simulink model "steering_validation"  (R2018b)
settings: Solver=VariableStepAuto  StartTime=0.0  StopTime=10.0  RelTol=1e-3
values from neighbouring files (symbols this model uses):
  D_steering_position = 0    [report_gutman.m]    (also in steering_extract_data.m)
  I_steering_position = 30    [report_gutman.m]    (also in steering_extract_data.m = 0)
  K_feedforward_steering = 0    [report_gutman.m]    (also in steering_extract_data.m)
  num_tf_steering = [253.4]    [report_gutman.m]    (also in steering_extract_data.m)
  P_steering_position = 30    [report_gutman.m]    (also in steering_extract_data.m)
  Ts = 0.01    [plot_poles.m]    (also in report_gutman.m; steering_extract_data.m)
libraries: simulink_extras x4, simulink x2
settings Model: Creator=maximef  LastModifiedBy=maximef

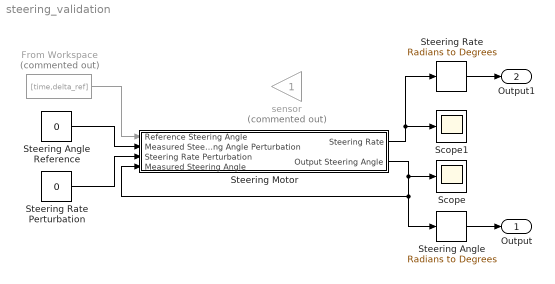
== system steering_validation ==
  From Workspace : FromWorkspace  Commented=on  VariableName=[time,delta_ref]  SampleTime=0
  Scope : Scope
  Scope1 : Scope
  Steering Angle : simulink_extras/Transformations/Radians to Degrees
  Steering Angle Reference : Constant  Value=0
  Steering Motor : Subsystem
  Steering Rate : simulink_extras/Transformations/Radians to Degrees
  Steering Rate Perturbation : Constant  Value=0
  sensor : Gain  Commented=on
  Output : Outport
  Output1 : Outport  Port=2
  wires:
  From Workspace/1 -> Steering Motor/1(Reference Steering Angle)
  Steering Motor/2(Output Steering Angle) -> Steering Angle/1, Steering Motor/4(Measured Steering Angle), Scope/1
  Steering Angle/1 -> Output/1
  Steering Rate Perturbation/1 -> Steering Motor/3(Steering Rate Perturbation)
  Steering Angle Reference/1 -> Steering Motor/2(Measured Steering Angle Perturbation)
  Steering Rate/1 -> Output1/1
  Steering Motor/1(Steering Rate) -> Scope1/1, Steering Rate/1

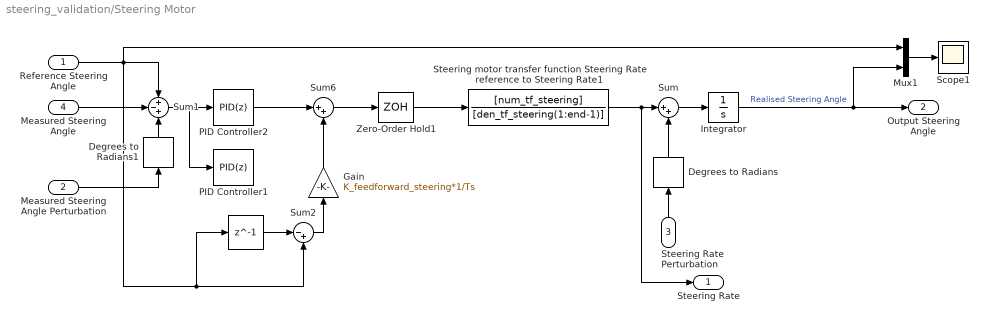
== system steering_validation/Steering Motor ==
  Reference Steering Angle : Inport
  Measured Steering Angle Perturbation : Inport  Port=2
  Steering Rate Perturbation : Inport  Port=3
  Measured Steering Angle : Inport  Port=4
  " " : Delay  DelayLength=1  SampleTime=Ts
  Degrees to Radians : simulink_extras/Transformations/Degrees to Radians
  Degrees to Radians1 : simulink_extras/Transformations/Degrees to Radians
  Gain : Gain  Gain=K_feedforward_steering*1/Ts
  Integrator : Integrator  InitialCondition=deg2rad(2)
  Mux1 : Mux  Inputs=2
  PID Controller1 : simulink/Continuous/PID Controller  Controller=PID  Form=Parallel  TimeDomain=Discrete-time  SampleTime=Ts  IntegratorMethod=Forward Euler  FilterMethod=Forward Euler  ControllerParametersSource=internal  P=P_steering_position  I=I_steering_position  D=D_steering_position  UseFilter=off  N=1  TunerSelectOption=Transfer Function Based (PID Tuner App)  InitialConditionSource=internal  InitialConditionForIntegrator=0  InitialConditionForFilter=0  DifferentiatorICPrevScaledInput=0  ExternalReset=none  TrackingMode=off  Kt=1  LimitOutput=off  UpperSaturationLimit=inf  LowerSaturationLimit=-inf  LinearizeAsGain=on  AntiWindupMode=none  Kb=1  POutMin=[]  POutMax=[]  IOutMin=[]  IOutMax=[]  DOutMin=[]  DOutMax=[]  NOutMin=[]  NOutMax=[]  SumOutMin=[]  SumOutMax=[]  SaturationOutMin=[]  SaturationOutMax=[]  PParamMin=[]  PParamMax=[]  IParamMin=[]  IParamMax=[]  DParamMin=[]  DParamMax=[]  NParamMin=[]  NParamMax=[]  KbParamMin=[]  KbParamMax=[]  KtParamMin=[]  KtParamMax=[]  KbOutMin=[]  KbOutMax=[]  KtOutMin=[]  KtOutMax=[]  IntegratorOutMin=[]  IntegratorOutMax=[]  FilterOutMin=[]  FilterOutMax=[]  SumI1OutMin=[]  SumI1OutMax=[]  SumI2OutMin=[]  SumI2OutMax=[]  SumI3OutMin=[]  SumI3OutMax=[]  SumI4OutMin=[]  SumI4OutMax=[]  SumDOutMin=[]  SumDOutMax=[]  DifferentiatorOutMin=[]  DifferentiatorOutMax=[]  FilterDiffOutCoefMin=[]  FilterDiffOutCoefMax=[]  ReciprocalOutMin=[]  ReciprocalOutMax=[]  SumDenOutMin=[]  SumDenOutMax=[]  SumNumOutMin=[]  SumNumOutMax=[]  DivideOutMin=[]  DivideOutMax=[]  IntegratorContinuousStateAttributes=''  IntegratorStateMustResolveToSignalObject=off  IntegratorRTWStateStorageClass=Auto  FilterContinuousStateAttributes=''  FilterStateMustResolveToSignalObject=off  FilterRTWStateStorageClass=Auto  ParallelPVariant=InternalParameters  IdealPVariant=Disabled  IVariant=InternalParameters  DVariant=InternalParameters  IntegratorVariant=Discrete  SatVariant=Disabled  AWVariant=Passthrough  PCopyVariant=Disabled  TRVariant=Disabled  FdbkBlocksVariant=Forward  IdealPFdbkVariant=Disabled  SatFdbkVariant=Disabled  DerivativeFilterVariant=Differentiator  NVariant=Passthrough  NCopyVariant=Disabled_SignalSpec  FilterICVariant=InternalICsDifferentiator  IntegratorICVariant=InternalICs  ExternalResetVariant=Disabled  TRSumVariant=Passthrough  SumFdbkVariant=Disabled  SumVariant=Sum_PID
  PID Controller2 : simulink/Continuous/PID Controller  Controller=PID  Form=Parallel  TimeDomain=Discrete-time  SampleTime=Ts  IntegratorMethod=Forward Euler  FilterMethod=Forward Euler  ControllerParametersSource=internal  P=0.1  I=0  D=0.04  UseFilter=off  N=1  TunerSelectOption=Transfer Function Based (PID Tuner App)  InitialConditionSource=internal  InitialConditionForIntegrator=0  InitialConditionForFilter=0  DifferentiatorICPrevScaledInput=0  ExternalReset=none  TrackingMode=off  Kt=1  LimitOutput=off  UpperSaturationLimit=inf  LowerSaturationLimit=-inf  LinearizeAsGain=on  AntiWindupMode=none  Kb=1  POutMin=[]  POutMax=[]  IOutMin=[]  IOutMax=[]  DOutMin=[]  DOutMax=[]  NOutMin=[]  NOutMax=[]  SumOutMin=[]  SumOutMax=[]  SaturationOutMin=[]  SaturationOutMax=[]  PParamMin=[]  PParamMax=[]  IParamMin=[]  IParamMax=[]  DParamMin=[]  DParamMax=[]  NParamMin=[]  NParamMax=[]  KbParamMin=[]  KbParamMax=[]  KtParamMin=[]  KtParamMax=[]  KbOutMin=[]  KbOutMax=[]  KtOutMin=[]  KtOutMax=[]  IntegratorOutMin=[]  IntegratorOutMax=[]  FilterOutMin=[]  FilterOutMax=[]  SumI1OutMin=[]  SumI1OutMax=[]  SumI2OutMin=[]  SumI2OutMax=[]  SumI3OutMin=[]  SumI3OutMax=[]  SumI4OutMin=[]  SumI4OutMax=[]  SumDOutMin=[]  SumDOutMax=[]  DifferentiatorOutMin=[]  DifferentiatorOutMax=[]  FilterDiffOutCoefMin=[]  FilterDiffOutCoefMax=[]  ReciprocalOutMin=[]  ReciprocalOutMax=[]  SumDenOutMin=[]  SumDenOutMax=[]  SumNumOutMin=[]  SumNumOutMax=[]  DivideOutMin=[]  DivideOutMax=[]  IntegratorContinuousStateAttributes=''  IntegratorStateMustResolveToSignalObject=off  IntegratorRTWStateStorageClass=Auto  FilterContinuousStateAttributes=''  FilterStateMustResolveToSignalObject=off  FilterRTWStateStorageClass=Auto  ParallelPVariant=InternalParameters  IdealPVariant=Disabled  IVariant=InternalParameters  DVariant=InternalParameters  IntegratorVariant=Discrete  SatVariant=Disabled  AWVariant=Passthrough  PCopyVariant=Disabled  TRVariant=Disabled  FdbkBlocksVariant=Forward  IdealPFdbkVariant=Disabled  SatFdbkVariant=Disabled  DerivativeFilterVariant=Differentiator  NVariant=Passthrough  NCopyVariant=Disabled_SignalSpec  FilterICVariant=InternalICsDifferentiator  IntegratorICVariant=InternalICs  ExternalResetVariant=Disabled  TRSumVariant=Passthrough  SumFdbkVariant=Disabled  SumVariant=Sum_PID
  Scope1 : Scope
  Steering motor transfer function Steering Rate reference to Steering Rate1 : TransferFcn  Numerator=[num_tf_steering]  Denominator=[den_tf_steering(1:end-1)]
  Sum : Sum  Inputs=|++
  Sum1 : Sum  Inputs=+-+
  Sum2 : Sum  Inputs=|-+
  Sum6 : Sum  Inputs=|++
  Zero-Order Hold1 : ZeroOrderHold  SampleTime=Ts
  Steering Rate : Outport
  Output Steering Angle : Outport  Port=2
  wires:
  Mux1/1 -> Scope1/1
  Sum6/1 -> Zero-Order Hold1/1
  Reference Steering Angle/1 -> Mux1/1, Sum1/1, Sum2/2, " "/1
  Measured Steering Angle/1 -> Sum1/2
  " "/1 -> Sum2/1
  Sum2/1 -> Gain/1
  Sum1/1 -> PID Controller2/1, PID Controller1/1
  Zero-Order Hold1/1 -> Steering motor transfer function Steering Rate reference to Steering Rate1/1
  Integrator/1 -> Output Steering Angle/1, Mux1/2  "Realised Steering Angle"
  Gain/1 -> Sum6/2
  Steering motor transfer function Steering Rate reference to Steering Rate1/1 -> Steering Rate/1, Sum/1
  Steering Rate Perturbation/1 -> Degrees to Radians/1
  Degrees to Radians/1 -> Sum/2
  Sum/1 -> Integrator/1
  Measured Steering Angle Perturbation/1 -> Degrees to Radians1/1
  Degrees to Radians1/1 -> Sum1/3
  PID Controller2/1 -> Sum6/1
